simulink model "MIAC_ZTransform"  (R2018b)
settings: Solver=FixedStepDiscrete  StartTime=0.0  StopTime=5.5*10^4  FixedStep=1  RelTol=1e-3
undefined symbols (not defined in the file or in its folder): sigbuilder_block
libraries: simulink x2, peGeneralControl x2, slident x1
settings Model: Creator=Trips  LastModifiedBy=Trips

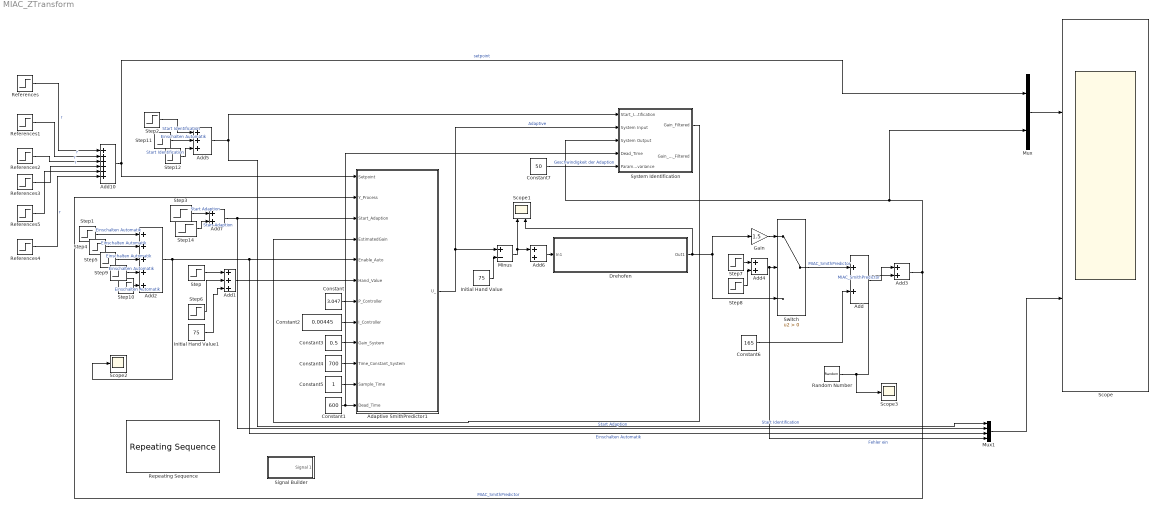
== system MIAC_ZTransform ==
  Adaptive SmithPredictor1 : Subsystem
  Add{,3..4,6..7} (5 alike) : Sum
  Add1 : Sum  Inputs=+++
  Add10 : Sum  Inputs=++++++
  Add2 : Sum  Inputs=5
  Add5 : Sum  Inputs=+++
  Constant : Constant  Value=3.047
  Constant1 : Constant  Value=600
  Constant2 : Constant  Value=0.00445
  Constant3 : Constant  Value=0.5
  Constant4 : Constant  Value=700
  Constant5 : Constant
  Constant6 : Constant  Value=165
  Constant7 : Constant  Value=50
  Drehofen : Subsystem
  Gain : Gain  Gain=1.5
  Initial Hand Value : Constant  Value=75
  Initial Hand Value1 : Constant  Value=75
  Minus : Sum  Inputs=+-
  Mux : Mux  Inputs=2
  Mux1 : Mux
  Random Number : RandomNumber  Variance=0.01  SampleTime=10
  References : Step  After=3
  References1 : Step  Time=12000  After=2
  References2 : Step  Time=18000  After=3
  References3 : Step  Time=35000  After=3
  References4 : Step  Time=0  After=165
  References5 : Step  Time=40000  After=-7
  Repeating Sequence : simulink/Sources/Repeating Sequence  rep_seq_t=[0 3999 4000 19999 20000 24999 25000]  rep_seq_y=[0 0 1 1 0 0 1]
  Scope : Scope  NumInputPorts=2
  Scope1 : Scope  NumInputPorts=2
  Scope2 : Scope
  Scope3 : Scope
  Signal Builder : Subsystem  Tag=STV Subsys  LoadFcn=sigbuilder_block('load');  StartFcn=sigbuilder_block('start');  StopFcn=sigbuilder_block('stop');  ClipboardFcn=sigbuilder_block('clipboard');  mask(Sigbuilder block){tuvar=[0:10]}
      mask help: Simulink:masks:SigbuilderBlock_MD
      mask init:
      | if ~strcmp(get_param(bdroot(gcbh),'SimulationStatus'),'stopped') tuvar = sigbuilder_block('maskInit'); end
      settings: CopyFcn=sigbuilder_block('copy');  DeleteFcn=sigbuilder_block('delete');  ModelCloseFcn=sigbuilder_block('modelClose');  PreSaveFcn=sigbuilder_block('preSave');  PauseFcn=sigbuilder_block('pause');  ContinueFcn=sigbuilder_block('continue');  NameChangeFcn=sigbuilder_block('namechange');  OpenFcn=sigbuilder_block('open',[437.6 199.2 550.4 400 ]);  CloseFcn=sigbuilder_block('close');
      mask Display: plot(0, 0, 100, 100,[2, 2, 32, 32, 2], [68, 8, 8, 68, 68],[32, 2], [38, 38], [32, 19, 2],[53, 60, 44], [32, 17, 17, 2],[16, 16, 31, 31]);txt = getActiveGroup(gcbh);text(2, 100, txt,'verticalAlignment', 'top');
  Step : Step  Time=300  After=5  SampleTime=0
  Step1 : Step  Time=4000  SampleTime=0
  Step10 : Step  Time=50000  SampleTime=0
  Step11 : Step  Time=35000  After=-1  SampleTime=0
  Step12 : Step  Time=38000  SampleTime=1
  Step14 : Step  Time=3*10^4  After=-1  SampleTime=1
  Step2 : Step  Time=3900  SampleTime=1
  Step3 : Step  Time=5000  Before=1  After=0  SampleTime=1
  Step4 : Step  Time=20000  After=-1  SampleTime=0
  Step5 : Step  Time=25000  SampleTime=0
  Step6 : Step  Time=19000  After=5  SampleTime=0
  Step7 : Step  Time=3*10^4  SampleTime=0
  Step8 : Step  Time=3.8*10^4  After=0  SampleTime=0
  Step9 : Step  Time=45000  After=-1  SampleTime=0
  Switch : Switch  Criteria=u2 > Threshold
  System Identification : Subsystem
  wires:
  Add3/1 -> Adaptive SmithPredictor1/2(Y_Process), System Identification/3(System Output), Mux/2  "MIAC_SmithPredictor"
  Add5/1 -> System Identification/1(Start_Identification), Mux1/1  "Start Identification"
  Adaptive SmithPredictor1/1(U_) -> System Identification/2(System Input), Minus/1  "Adaptive"
  References/1 -> Add10/1  "r"
  References2/1 -> Add10/3  "r"
  References3/1 -> Add10/4  "r"
  References1/1 -> Add10/2  "r"
  Add10/1 -> Adaptive SmithPredictor1/1(Setpoint), Mux/1  "setpoint"
  Add1/1 -> Adaptive SmithPredictor1/6(Hand_Value)
  Add2/1 -> Scope2/1, Adaptive SmithPredictor1/5(Enable_Auto), Mux1/3  "Einschalten Automatik"
  Constant/1 -> Adaptive SmithPredictor1/7(P_Controller)
  Constant2/1 -> Adaptive SmithPredictor1/8(I_Controller)
  Constant3/1 -> Adaptive SmithPredictor1/9(Gain_System)
  Constant4/1 -> Adaptive SmithPredictor1/10(Time_Constant_System)
  Constant5/1 -> Adaptive SmithPredictor1/11(Sample_Time)
  Constant1/1 -> System Identification/4(Dead_Time), Adaptive SmithPredictor1/12(" Dead_Time")
  System Identification/1(Gain_Filtered) -> Adaptive SmithPredictor1/4(EstimatedGain)
  References4/1 -> Add10/6  "r"
  Minus/1 -> Add6/1, Scope1/1
  Constant6/1 -> Add/2
  Mux1/1 -> Scope/2
  Mux/1 -> Scope/1
  Initial Hand Value/1 -> Minus/2
  Step/1 -> Add1/1
  Initial Hand Value1/1 -> Add1/3
  Step1/1 -> Add2/1  "Einschalten Automatik"
  Step4/1 -> Add2/2  "Einschalten Automatik"
  Step5/1 -> Add2/3  "Einschalten Automatik"
  Step6/1 -> Add1/2
  Add/1 -> Add3/1  "MIAC_SmithPredictor"
  Random Number/1 -> Scope3/1, Add3/2
  Step7/1 -> Add4/1
  Drehofen/1(Out1) -> Scope1/2, Gain/1, Switch/3
  Switch/1 -> Add/1  "MIAC_SmithPredictor"
  Add4/1 -> Switch/2, Mux1/4  "Fehler ein"
  Step8/1 -> Add4/2
  References5/1 -> Add10/5
  Gain/1 -> Switch/1
  Step10/1 -> Add2/5  "Einschalten Automatik"
  Step9/1 -> Add2/4  "Einschalten Automatik"
  Add7/1 -> Mux1/2, Adaptive SmithPredictor1/3(Start_Adaption)  "Start Adaption"
  Step11/1 -> Add5/2  "Einschalten Automatik"
  Step2/1 -> Add5/1  "Start Identification"
  Step12/1 -> Add5/3  "Start Identification"
  Add6/1 -> Drehofen/1(In1)
  Step3/1 -> Add7/1  "Start Adaption"
  Step14/1 -> Add7/2  "Start Adaption"
  Constant7/1 -> System Identification/5(Parameter_Covariance)  "Geschwindigkeit der Adaption"

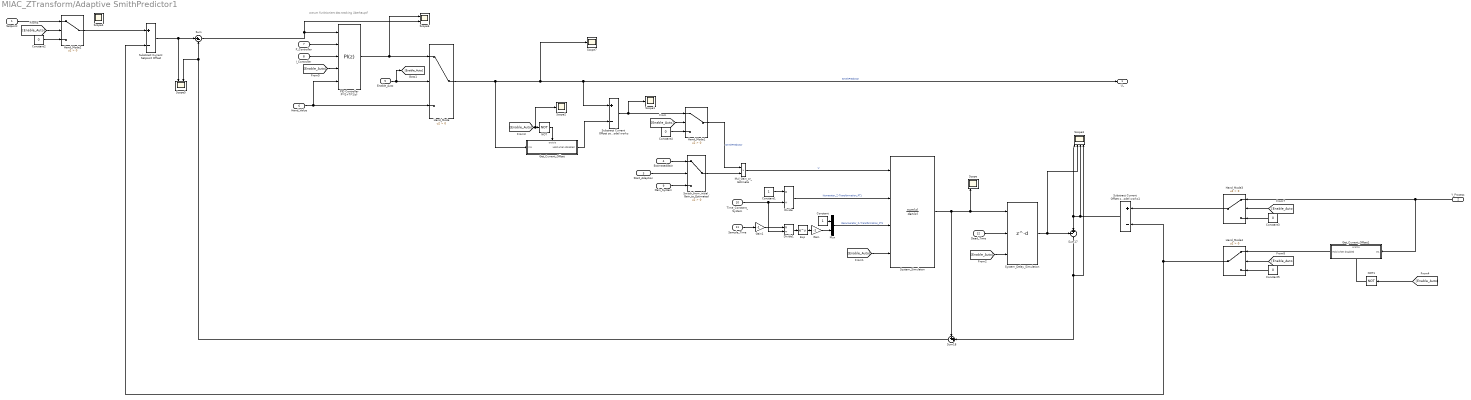
== system MIAC_ZTransform/Adaptive SmithPredictor1 ==
  note: warum funktioniert das tracking überhaupt?
  Setpoint : Inport
  Y_Process : Inport  Port=2
  Start_Adaption : Inport  Port=3
  EstimatedGain : Inport  Port=4
  Enable_Auto : Inport  Port=5
  Hand_Value : Inport  Port=6
  P_Controller : Inport  Port=7
  I_Controller : Inport  Port=8
  Gain_System : Inport  Port=9
  Time_Constant_System : Inport  Port=10
  Sample_Time : Inport  Port=11
  " Dead_Time" : Inport  Port=12
  Constant : Constant
  Constant1 : Constant
  Constant{2..5} (4 alike) : Constant  Value=0
  Divide : Product  Inputs=*/
  Divide1 : Product  Inputs=*/
  Exp : Math  SaturateOnIntegerOverflow=on
  Gain : Gain  Gain=-1
  Gain1 : Gain  Gain=-1
  Get_Current_Offset : Subsystem
  Get_Current_Offset1 : Subsystem
  Hand_Mode{,1..4} (5 alike) : Switch  Criteria=u2 > Threshold
  Mul_Gain_or_Estimate : Product
  Mux : Mux  Inputs=2
  NOT : Logic  Operator=NOT  IconShape=distinctive  AllPortsSameDT=off  OutDataTypeStr=boolean
  NOT1 : Logic  Operator=NOT  IconShape=distinctive  AllPortsSameDT=off  OutDataTypeStr=boolean
  PID Controller P*(1+Ti*1/s) : simulink/Continuous/PID Controller  Controller=PI  Form=Parallel  TimeDomain=Discrete-time  SampleTime=1  IntegratorMethod=Forward Euler  FilterMethod=Forward Euler  ControllerParametersSource=external  P=3.04732259067536  I=0.00445689106465138  D=118.272348286844  UseFilter=on  N=0.00420306193364532  TunerSelectOption=Transfer Function Based (PID Tuner App)  InitialConditionSource=external  InitialConditionForIntegrator=0  InitialConditionForFilter=0  DifferentiatorICPrevScaledInput=0  ExternalReset=rising  TrackingMode=off  Kt=1  LimitOutput=on  UpperSaturationLimit=100  LowerSaturationLimit=0  LinearizeAsGain=on  AntiWindupMode=none  Kb=1  POutMin=[]  POutMax=[]  IOutMin=[]  IOutMax=[]  DOutMin=[]  DOutMax=[]  NOutMin=[]  NOutMax=[]  SumOutMin=[]  SumOutMax=[]  SaturationOutMin=[]  SaturationOutMax=[]  PParamMin=[]  PParamMax=[]  IParamMin=[]  IParamMax=[]  DParamMin=[]  DParamMax=[]  NParamMin=[]  NParamMax=[]  KbParamMin=[]  KbParamMax=[]  KtParamMin=[]  KtParamMax=[]  KbOutMin=[]  KbOutMax=[]  KtOutMin=[]  KtOutMax=[]  IntegratorOutMin=[]  IntegratorOutMax=[]  FilterOutMin=[]  FilterOutMax=[]  SumI1OutMin=[]  SumI1OutMax=[]  SumI2OutMin=[]  SumI2OutMax=[]  SumI3OutMin=[]  SumI3OutMax=[]  SumI4OutMin=[]  SumI4OutMax=[]  SumDOutMin=[]  SumDOutMax=[]  DifferentiatorOutMin=[]  DifferentiatorOutMax=[]  FilterDiffOutCoefMin=[]  FilterDiffOutCoefMax=[]  ReciprocalOutMin=[]  ReciprocalOutMax=[]  SumDenOutMin=[]  SumDenOutMax=[]  SumNumOutMin=[]  SumNumOutMax=[]  DivideOutMin=[]  DivideOutMax=[]  IntegratorContinuousStateAttributes=''  IntegratorStateMustResolveToSignalObject=off  IntegratorRTWStateStorageClass=Auto  FilterContinuousStateAttributes=''  FilterStateMustResolveToSignalObject=off  FilterRTWStateStorageClass=Auto  ParallelPVariant=ExternalParameters  IdealPVariant=Disabled  IVariant=ExternalParameters  DVariant=Disabled  IntegratorVariant=Discrete  SatVariant=Enabled  AWVariant=Passthrough  PCopyVariant=Disabled  TRVariant=Disabled  FdbkBlocksVariant=Forward  IdealPFdbkVariant=Disabled  SatFdbkVariant=Disabled  DerivativeFilterVariant=Disabled  NVariant=Disabled  NCopyVariant=Disabled_SignalSpec  FilterICVariant=Disabled  IntegratorICVariant=ExternalICs  ExternalResetVariant=ExternalReset  TRSumVariant=Passthrough  SumFdbkVariant=Disabled  SumVariant=Sum_PI
  Scope : Scope  NumInputPorts=3
  Scope{1..2,4,7} (4 alike) : Scope
  Scope3 : Scope  NumInputPorts=4
  Scope5 : Scope  NumInputPorts=2
  Scope6 : Scope  NumInputPorts=2
  Substract Current Offset so that the linearised model works : Sum  Inputs=+-
  Substract Current Offset so that the linearised model works1 : Sum  Inputs=+-
  Substract Current Setpoint Offset : Sum  Inputs=+-
  Sum : Sum  Inputs=|+-
  Sum17 : Sum  Inputs=-+|
  Sum18 : Sum  Inputs=++|
  Switch_from_initial_Gain_to_Estimated : Switch  Criteria=u2 > Threshold
  System_Delay_Simulation : Delay  DelayLengthSource=Input port  DelayLength=600  DelayLengthUpperLimit=800  ExternalReset=Rising  SampleTime=1
      settings: InputPortMap=u0,p1,r5
  System_Simulaton : DiscreteTransferFcn  NumeratorSource=Input port  DenominatorSource=Input port  ExternalReset=Rising  SampleTime=1  a0EqualsOne=on
      settings: InputPortMap=u0,p1,p3,r7
  U_ : Outport
  wires:
  Substract Current Setpoint Offset/1 -> Scope5/1, Sum/1
  Sum/1 -> Scope6/2, PID Controller P*(1+Ti*1/s)/1
  Hand_Mode/1 -> Scope7/1, U_/1, Substract Current Offset so that the linearised model works/1, Get_Current_Offset/1(In1)  "SmithPredictor"
  Substract Current Offset so that the linearised model works1/1 -> Scope3/3, Sum17/2, Scope3/1
  System_Simulaton/1 -> Sum18/1, Scope/1, System_Delay_Simulation/1
  System_Delay_Simulation/1 -> Scope3/2, Sum17/1
  Sum17/1 -> Scope3/4, Sum18/2
  Mul_Gain_or_Estimate/1 -> System_Simulaton/1  "U"
  Switch_from_initial_Gain_to_Estimated/1 -> Mul_Gain_or_Estimate/2
  PID Controller P*(1+Ti*1/s)/1 -> Scope6/1, Hand_Mode/1
  Hand_Value/1 -> PID Controller P*(1+Ti*1/s)/5, Hand_Mode/3
  Enable_Auto/1 -> [Enable_Auto], Hand_Mode/2
  P_Controller/1 -> PID Controller P*(1+Ti*1/s)/2
  I_Controller/1 -> PID Controller P*(1+Ti*1/s)/3
  Divide/1 -> System_Simulaton/2  "Numerator_Z-Transformation_PT1"
  Mux/1 -> System_Simulaton/3  "Denumerator_Z-Transformation_PT1"
  Time_Constant_System/1 -> Divide1/2, Divide/2
  Constant/1 -> Mux/1
  Exp/1 -> Gain/1
  Gain/1 -> Mux/2
  Divide1/1 -> Exp/1
  Sample_Time/1 -> Gain1/1
  " Dead_Time"/1 -> System_Delay_Simulation/2
  Gain_System/1 -> Switch_from_initial_Gain_to_Estimated/3
  Start_Adaption/1 -> Switch_from_initial_Gain_to_Estimated/2
  EstimatedGain/1 -> Switch_from_initial_Gain_to_Estimated/1
  Constant1/1 -> Divide/1
  Gain1/1 -> Divide1/1
  [Enable_Auto] -> Hand_Mode1/2
  Hand_Mode1/1 -> Mul_Gain_or_Estimate/1  "SmithPredictor"
  Constant4/1 -> Hand_Mode1/3
  [Enable_Auto] -> System_Simulaton/4
  [Enable_Auto] -> System_Delay_Simulation/3
  Substract Current Offset so that the linearised model works/1 -> Scope1/1, Hand_Mode1/1
  Get_Current_Offset/1(Hold when disabled) -> Substract Current Offset so that the linearised model works/2
  [Enable_Auto] -> Scope2/1, NOT/1
  NOT/1 -> Get_Current_Offset/Enable
  Sum18/1 -> Scope5/2, Sum/2
  Hand_Mode2/1 -> Substract Current Setpoint Offset/1
  NOT1/1 -> Get_Current_Offset1/Enable
  [Enable_Auto] -> NOT1/1
  Hand_Mode4/1 -> Substract Current Setpoint Offset/2, Substract Current Offset so that the linearised model works1/2
  [Enable_Auto] -> PID Controller P*(1+Ti*1/s)/4
  Setpoint/1 -> Hand_Mode2/1
  [Enable_Auto] -> Hand_Mode2/2
  Constant2/1 -> Hand_Mode2/3
  Y_Process/1 -> Get_Current_Offset1/1(In1), Hand_Mode3/1
  [Enable_Auto] -> Hand_Mode3/2
  Constant3/1 -> Hand_Mode3/3
  Hand_Mode3/1 -> Substract Current Offset so that the linearised model works1/1
  Constant5/1 -> Hand_Mode4/3
  [Enable_Auto] -> Hand_Mode4/2
  Get_Current_Offset1/1(Hold when disabled) -> Hand_Mode4/1

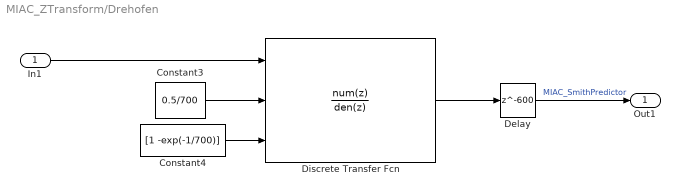
== system MIAC_ZTransform/Drehofen ==
  In1 : Inport
  Constant3 : Constant  Value=0.5/700
  Constant4 : Constant  Value=[1 -exp(-1/700)]
  Delay : Delay  DelayLength=600
  Discrete Transfer Fcn : DiscreteTransferFcn  NumeratorSource=Input port  DenominatorSource=Input port  a0EqualsOne=on
      settings: InputPortMap=u0,p1,p3
  Out1 : Outport
  wires:
  Discrete Transfer Fcn/1 -> Delay/1
  Constant4/1 -> Discrete Transfer Fcn/3
  Constant3/1 -> Discrete Transfer Fcn/2
  In1/1 -> Discrete Transfer Fcn/1
  Delay/1 -> Out1/1  "MIAC_SmithPredictor"

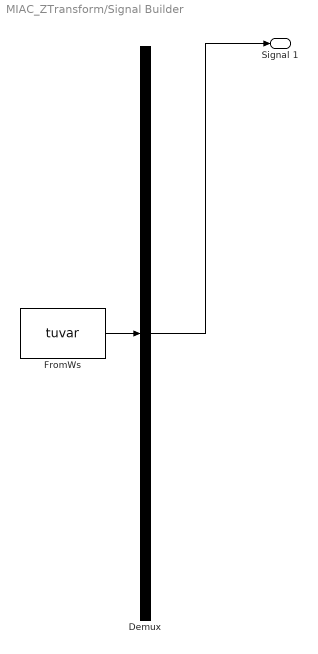
== system MIAC_ZTransform/Signal Builder ==
  Demux : Demux  Tag=STV Demux  Outputs=1
  FromWs : FromWorkspace  Tag=STV FromWs  VariableName=tuvar  SampleTime=0
      SigBuilderData=|
      | common.afterFinalStr = 'Extrapolate'
      | common.sampleTime = 0
      | dataSet.timeRange = [0 55000]
      | dataSet.name = 'Group 1'
      | sbobj.Groups.Name = 'Group 1'
      | sbobj.Groups.Signals.Name = 'Signal 1'
      | sbobj.Groups.Signals.XData = [0 4 4 55000]
      | sbobj.Groups.Signals.YData = [0 0 1 1]
      | sbobj.Groups.TimeRange = [0 55000]
  Signal 1 : Outport  Tag=STV Outport
  wires:
  Demux/1 -> Signal 1/1
  FromWs/1 -> Demux/1

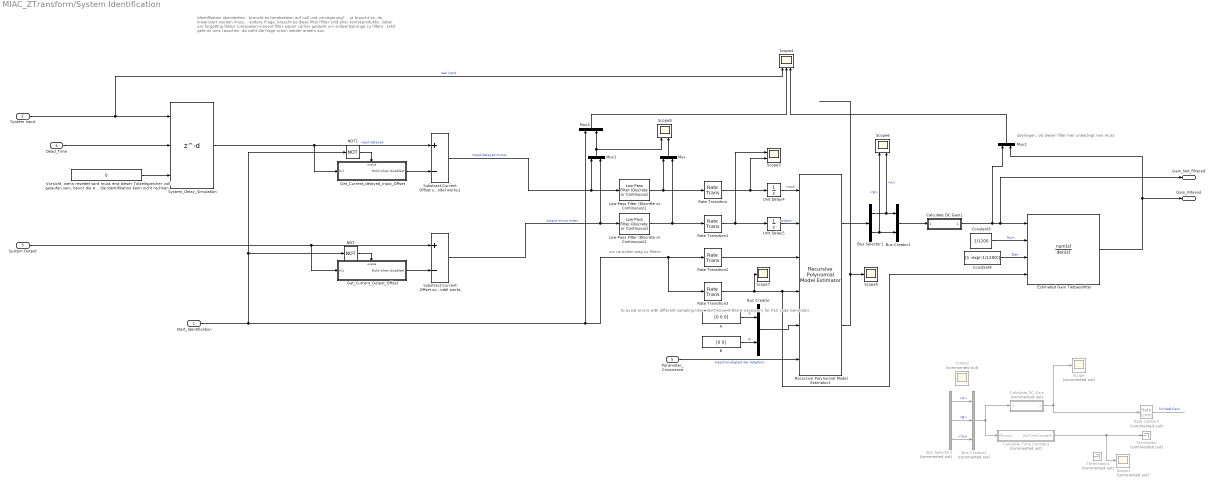
== system MIAC_ZTransform/System Identification ==
  note: um rauschen weg zu filtern
  note: überlegen, ob dieser filter hier unbedingt rein muss
  note: Identifikation überdenken...braucht es herabsetzen auf null und verzögerung?
      | ...ja braucht es, da linearisiert werden muss...
      |
      | andere Frage, braucht es diese filter?filter sind eher kontraproduktiv, lieber am forgetting faktor rumspielen
      | monent fliter waren vorher gedacht um sollwertsprünge zu filtern...jetzt geht es ums rauschen, da sieht die frage schon weider anders aus
  note: to avoid errors with different sampling time, don't know if this is necessary for PLC code Generator
  Start_Identification : Inport
  System Input : Inport  Port=2
  System Output : Inport  Port=3
  Dead_Time : Inport  Port=4
  Parameter_Covariance : Inport  Port=5
  A : Constant  Value=[0 0 0]  VectorParams1D=off
  B : Constant  Value=[0 0]  VectorParams1D=off
  Bus Creator : BusCreator  Inputs=2
  Bus Creator1 : BusCreator  Inputs=2
  Bus Creator2 : BusCreator  Commented=on  Inputs=3
  Bus Selector1 : BusSelector  OutputSignals=A,B
  Bus Selector2 : BusSelector  Commented=on  OutputSignals=A,B,Ts
  Calculate DC Gain : Subsystem  Commented=on
  Calculate DC Gain1 : Subsystem
  Calculate Time Constant : Subsystem  Commented=on
  Constant3 : Constant  Value=1/1200
  Constant4 : Constant  Value=[1 -exp(-1/1200)]
  Estimated Gain Tiefpassfilter : DiscreteTransferFcn  NumeratorSource=Input port  DenominatorSource=Input port  ExternalReset=Rising  a0EqualsOne=on
      settings: InputPortMap=u0,p1,p3,r7
  Get_Current_Output_Offset : Subsystem
  Get_Current_delayed_Input_Offset : Subsystem
  Low-Pass Filter (Discrete or Continuous)1 : peGeneralControl/Low-Pass Filter (Discrete or Continuous)  K=1  T=100  B=inf  A=-inf  Ts=-1
  Low-Pass Filter (Discrete or Continuous)2 : peGeneralControl/Low-Pass Filter (Discrete or Continuous)  K=1  T=100  B=inf  A=-inf  Ts=-1
  Mux{,1..3} (4 alike) : Mux  Inputs=2
  NOT : Logic  Operator=NOT  IconShape=distinctive  AllPortsSameDT=off  OutDataTypeStr=boolean
  NOT1 : Logic  Operator=NOT  IconShape=distinctive  AllPortsSameDT=off  OutDataTypeStr=boolean
  Rate Limiter2 : RateLimiter  Commented=on  SampleTimeMode=inherited
  Rate Transition{,1..3} (4 alike) : RateTransition  OutPortSampleTime=1
  Recursive Polynomial Model Estimator1 : slident/Estimators/Recursive Polynomial Model Estimator  ModelStructure=ARX  InitialEstimateSource=External  A0=2  B0=1  C0=1  D0=1  F0=1  nk=1  P0=100  InitialInputs=0  InitialOutputs=0  History=Infinite  WindowLength=2000  EstimationMethod=Forgetting Factor  AdaptationParameter=1  HasTimeVaryingAdaptationParameter=off  NormalizationBias=eps  OutputError=on  OutputP=off  AddEnablePort=on  ExternalReset=Rising  InputProcessing=Sample-based  Ts=1
      settings: SourceProductName=System Identification Toolbox  SourceProductBaseCode=ID
  Scope : Scope  Commented=on
  Scope1 : Scope  Commented=on
  Scope2 : Scope  Commented=on
  Scope3 : Scope  NumInputPorts=2
  Scope4 : Scope  NumInputPorts=3
  Scope5 : Scope
  Scope6 : Scope  NumInputPorts=2
  Scope7 : Scope
  Scope8 : Scope  NumInputPorts=2
  Substract Current Offset so that the linearised model works : Sum  Inputs=+-
  Substract Current Offset so that the linearised model works1 : Sum  Inputs=+-
  System_Delay_Simulation : Delay  DelayLengthSource=Input port  DelayLength=600  DelayLengthUpperLimit=800  ExternalReset=Rising  SampleTime=1
      settings: InputPortMap=u0,p1,r5
  Terminator : Terminator  Commented=on
  Terminator1 : Terminator  Commented=on
  Unit Delay4 : UnitDelay  InitialCondition=[0]
  Unit Delay5 : UnitDelay
  "Vorsicht, wenn resettet wird muss erst dieser Totzeitspeicher voll gelaufen sein, bevor die Adaption starten darf! Sonst kommt heir immer 0 raus und die Identifikation kann nicht rechnen." : Constant  Value=0
  Gain_Filtered : Outport
  Gain_Not_Filtered : Outport  Port=2
  wires:
  Recursive Polynomial Model Estimator1/1 -> Bus Selector1/1
  Unit Delay4/1 -> Recursive Polynomial Model Estimator1/1  "input"
  Unit Delay5/1 -> Recursive Polynomial Model Estimator1/2  "output"
  Rate Transition/1 -> Scope3/2, Unit Delay4/1
  Rate Transition1/1 -> Scope3/1, Unit Delay5/1
  Bus Selector2/3 -> Bus Creator2/3  "<Ts>"
  ? -> Bus Selector2/1
  Bus Selector2/1 -> Bus Creator2/1  "<A>"
  Calculate DC Gain/1(DCGain) -> Rate Limiter2/1, Scope/1
  Bus Creator2/1 -> Calculate DC Gain/1(Params), Calculate Time Constant/1(Params)
  Rate Limiter2/1 -> ?  "limited Gain"
  ? -> Terminator1/1
  ? -> Scope2/1
  Bus Selector2/2 -> Bus Creator2/2  "<B>"
  Calculate Time Constant/1("OutTimeConstant ") -> Scope1/1, Terminator/1
  Bus Creator1/1 -> Calculate DC Gain1/1(Params)
  Bus Selector1/1 -> Scope6/2, Bus Creator1/1  "<A>"
  Bus Selector1/2 -> Scope6/1, Bus Creator1/2  "<B>"
  Rate Transition2/1 -> Recursive Polynomial Model Estimator1/3
  Rate Transition3/1 -> Recursive Polynomial Model Estimator1/4, Estimated Gain Tiefpassfilter/4, Scope7/1
  Substract Current Offset so that the linearised model works/1 -> Low-Pass Filter (Discrete or Continuous)2/1, Mux1/2  "output minus mean"
  NOT/1 -> Get_Current_Output_Offset/Enable
  Get_Current_Output_Offset/1(Hold when disabled) -> Substract Current Offset so that the linearised model works/2
  System Output/1 -> Get_Current_Output_Offset/1(In1), Substract Current Offset so that the linearised model works/1
  Get_Current_delayed_Input_Offset/1(Hold when disabled) -> Substract Current Offset so that the linearised model works1/2
  NOT1/1 -> Get_Current_delayed_Input_Offset/Enable
  Mux/1 -> Scope8/2
  Mux1/1 -> Mux3/2, Scope8/1
  Recursive Polynomial Model Estimator1/2 -> Scope5/1
  Start_Identification/1 -> NOT/1, NOT1/1, Rate Transition3/1, Rate Transition2/1, Mux3/1
  Mux3/1 -> Scope4/2
  Mux2/1 -> Scope4/3
  Estimated Gain Tiefpassfilter/1 -> Mux2/2, Gain_Filtered/1
  Low-Pass Filter (Discrete or Continuous)1/1 -> Rate Transition/1, Mux/1
  Low-Pass Filter (Discrete or Continuous)2/1 -> Rate Transition1/1, Mux/2
  System Input/1 -> Scope4/1, System_Delay_Simulation/1  "real input"
  "Vorsicht, wenn resettet wird muss erst dieser Totzeitspeicher voll gelaufen sein, bevor die Adaption starten darf! Sonst kommt heir immer 0 raus und die Identifikation kann nicht rechnen."/1 -> System_Delay_Simulation/3
  Dead_Time/1 -> System_Delay_Simulation/2
  Substract Current Offset so that the linearised model works1/1 -> Mux1/1, Low-Pass Filter (Discrete or Continuous)1/1  "imput delayed minus"
  System_Delay_Simulation/1 -> Substract Current Offset so that the linearised model works1/1, Get_Current_delayed_Input_Offset/1(In1)  "input delayed"
  Calculate DC Gain1/1(DCGain) -> Gain_Not_Filtered/1, Estimated Gain Tiefpassfilter/1, Mux2/1
  Constant3/1 -> Estimated Gain Tiefpassfilter/2  "Num"
  Constant4/1 -> Estimated Gain Tiefpassfilter/3  "Den"
  Parameter_Covariance/1 -> Recursive Polynomial Model Estimator1/6  "Geschwindigkeit der Adaption"
  Bus Creator/1 -> Recursive Polynomial Model Estimator1/5
  A/1 -> Bus Creator/1  "A"
  B/1 -> Bus Creator/2  "B"

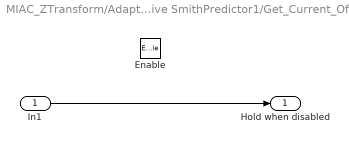
== system MIAC_ZTransform/Adaptive SmithPredictor1/Get_Current_Offset ==
  In1 : Inport
  Enable : EnablePort
  Hold when disabled : Outport
  wires:
  In1/1 -> Hold when disabled/1

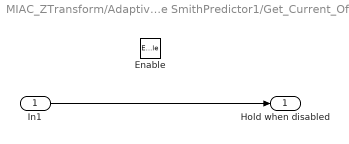
== system MIAC_ZTransform/Adaptive SmithPredictor1/Get_Current_Offset1 ==
  In1 : Inport
  Enable : EnablePort
  Hold when disabled : Outport
  wires:
  In1/1 -> Hold when disabled/1

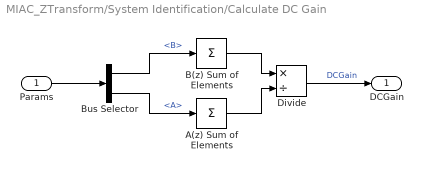
== system MIAC_ZTransform/System Identification/Calculate DC Gain ==
  Params : Inport
  A(z) Sum of Elements : Sum  Inputs=+
  B(z) Sum of Elements : Sum  Inputs=+
  Bus Selector : BusSelector  OutputSignals=B,A
  Divide : Product  Inputs=*/
  DCGain : Outport
  wires:
  A(z) Sum of Elements/1 -> Divide/2
  B(z) Sum of Elements/1 -> Divide/1
  Params/1 -> Bus Selector/1
  Bus Selector/1 -> B(z) Sum of Elements/1  "<B>"
  Bus Selector/2 -> A(z) Sum of Elements/1  "<A>"
  Divide/1 -> DCGain/1  "DCGain"

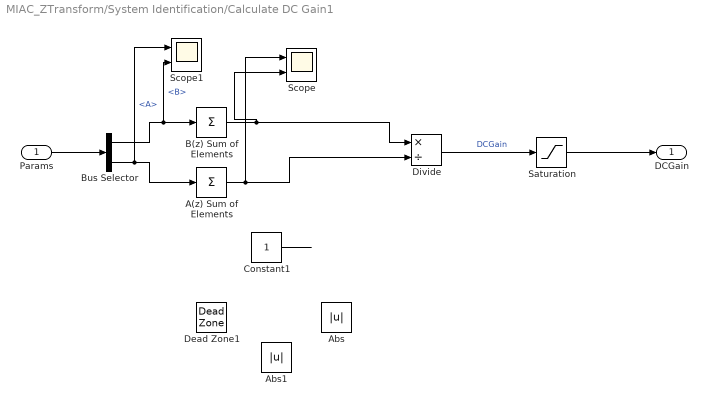
== system MIAC_ZTransform/System Identification/Calculate DC Gain1 ==
  Params : Inport
  A(z) Sum of Elements : Sum  Inputs=+
  Abs : Abs
  Abs1 : Abs
  B(z) Sum of Elements : Sum  Inputs=+
  Bus Selector : BusSelector  OutputSignals=B,A
  Constant1 : Constant
  Dead Zone1 : DeadZone  LowerValue=-0.001  UpperValue=0.001  SaturateOnIntegerOverflow=on
  Divide : Product  Inputs=*/
  Saturation : Saturate  UpperLimit=1.5  LowerLimit=0.01
  Scope : Scope  NumInputPorts=2
  Scope1 : Scope  NumInputPorts=2
  DCGain : Outport
  wires:
  Params/1 -> Bus Selector/1
  Bus Selector/1 -> Scope1/2, B(z) Sum of Elements/1  "<B>"
  Bus Selector/2 -> Scope1/1, A(z) Sum of Elements/1  "<A>"
  B(z) Sum of Elements/1 -> Divide/1, Scope/2
  Constant1/1 -> ?
  Divide/1 -> Saturation/1  "DCGain"
  A(z) Sum of Elements/1 -> Divide/2, Scope/1
  Saturation/1 -> DCGain/1

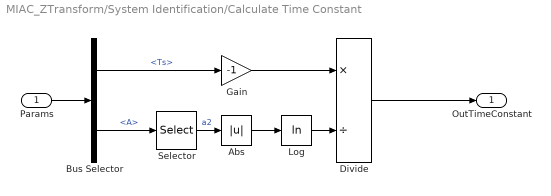
== system MIAC_ZTransform/System Identification/Calculate Time Constant ==
  Params : Inport
  Abs : Abs
  Bus Selector : BusSelector  OutputSignals=Ts,A
  Divide : Product  Inputs=*/
  Gain : Gain  Gain=-1
  Log : Math  Operator=log  SaturateOnIntegerOverflow=on
  Selector : Selector  InputPortWidth=2  IndexOptions=Starting index (dialog)  Indices=[2]  OutputSizes=1
  "OutTimeConstant " : Outport
  wires:
  Params/1 -> Bus Selector/1
  Bus Selector/1 -> Gain/1  "<Ts>"
  Bus Selector/2 -> Selector/1  "<A>"
  Selector/1 -> Abs/1  "a2"
  Gain/1 -> Divide/1
  Log/1 -> Divide/2
  Divide/1 -> "OutTimeConstant "/1
  Abs/1 -> Log/1

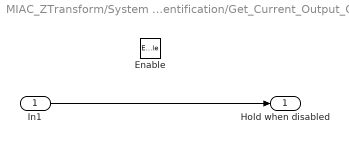
== system MIAC_ZTransform/System Identification/Get_Current_Output_Offset ==
  In1 : Inport
  Enable : EnablePort
  Hold when disabled : Outport
  wires:
  In1/1 -> Hold when disabled/1

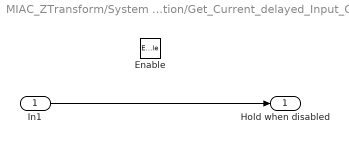
== system MIAC_ZTransform/System Identification/Get_Current_delayed_Input_Offset ==
  In1 : Inport
  Enable : EnablePort
  Hold when disabled : Outport
  wires:
  In1/1 -> Hold when disabled/1
